simulink model "gpsnoise"  (Simulink 3.00)
settings: Solver=ode45  StartTime=0.0  StopTime=500.0  RelTol=1e-3
libraries: simulink3 x4
settings Model: BooleanDataType=on  RTWOptions="-aEnforceIntegerDowncast=1 -aFoldNonRolledExpr=1 -aInlineInvariantSignals=1 -aInlineParameters=0 -aLocalBlockOutputs=1 -aRollThreshold=5 -aZeroInternalMemoryAtStartup=1 -aZeroExternalMemoryAtStartup=1 -aInitFltsAndDblsToZero=1 -aGenerateReport=0 -aGenCodeOnly=0 -aRTWVerbose=1 -aIncludeHyperlinkInReport=0 -aLaunchReport=0 -aForceParamTrailComments=0 -aGenerateComments=1 -aIgnoreCustomStorageClasses=1 -aIncHierarchyInIds=0 -aMaxRTWIdLen=31 -aShowEliminatedStatements=0 -aPrefixModelToSubsysFcnNames=1 -aIncDataTypeInIds=0 -aInsertBlockDesc=0 -aSimulinkBlockComments=1 -aInlinedPrmAccess=\"Literals\"  -aSuppressErrorStatus=0 -aModelReferenceCompliant=1 -aSupportNonInlinedSFcns=1 -aSupportContinuousTime=1 -aSupportComplex=1 -aSupportNonFinite=1 -aSupportAbsoluteTime=1 -aTargetFcnLib=\"ansi_tfl_tmw.mat\" -aMultiInstanceERTCode=0 -aLogVarNameModifier=\"rt_\" -aIsPILTarget=0 -aCombineOutputUpdateFcns=0 -aGenerateASAP2=0 -aGenerateSampleERTMain=0 -aGenerateFullHeader=1 -aUtilityFuncGeneration=\"Auto\" -aIncludeFileDelimiter=\"Auto\" -aIncludeMdlTerminateFcn=1 -aPurelyIntegerCode=0 -aERTCustomFileBanners=0 -aRTWCAPIStates=0 -aRTWCAPIParams=0 -aRTWCAPISignals=0 -aMatFileLogging=1 -aGenFloatMathFcnCalls=\"ANSI_C\" -aExtModeMexFile=\"ext_comm\" -aExtModeTransport=0 -aExtModeStaticAllocSize=1000000 -aExtModeTesting=0 -aExtModeStaticAlloc=0 -aExtMode=0"  ExtModeTrigMode=normal  ExtModeArmWhenConnect=on  LastModifiedBy=campa

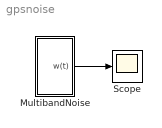
== system gpsnoise ==
  MultibandNoise : Subsystem  mask(Multiband Noise){n=3, power=[2e-5 0.01 0.2 2], time=[0.05 1 10 200], a=2, sd=3587, STime=0.1}
      mask prompts: n "Number Of Channels"; power "Noise Powers"; time "Sample Times (sec)"; a "Filter Cutoff Frequency (rad/sec)"; sd "Base Seed"; STime "Output Sampling Time"
      mask help:
      | This block models multiband noise using four different band limited
      |  white noise blocks, each one with its own power and time scale.
      |  A first order lowpass filter with a selectable cut off frequency is
      |  applied to the last three noises (have a look under the mask).
      |  The output sampling time has to be multiple of the first sample time.
      mask init:
      | n=fix(n);
      | T=time(1);T1=time(2);T2=time(3);T3=time(4);
      | P=power(1);P1=power(2);P2=power(3);P3=power(4);
      mask Help:
      | This block models multiband noise using four different band limited
      |  white noise blocks, each one with its own power and time scale.
      |  A first order lowpass filter with a selectable cut off frequency is
      |  applied to the last three noises (have a look under the mask).
      |  The output sampling time has to be multiple of the first sample time.
  Scope : Scope
      settings: TimeRange=500  YMin=-1  YMax=1  SaveToWorkspace=off  SaveName=ScopeData
  wires:
  MultibandNoise/1(w(t)) -> Scope/1

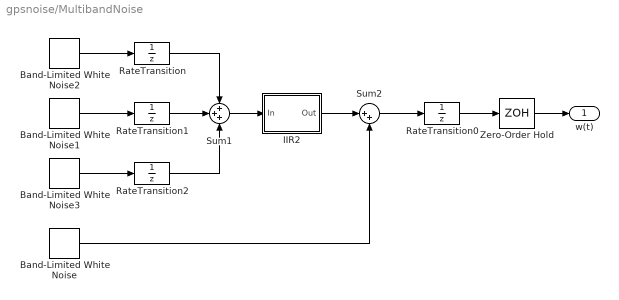
== system gpsnoise/MultibandNoise ==
  Band-Limited White Noise : simulink3/Sources/Band-Limited White Noise  Cov=P*ones(n,1)  Ts=T  seed=sd+[1:n]+0*n
  Band-Limited White Noise1 : simulink3/Sources/Band-Limited White Noise  Cov=P2*ones(n,1)  Ts=T2  seed=sd+[1:n]+2*n
  Band-Limited White Noise2 : simulink3/Sources/Band-Limited White Noise  Cov=P3*ones(n,1)  Ts=T3  seed=sd+[1:n]+1*n
  Band-Limited White Noise3 : simulink3/Sources/Band-Limited White Noise  Cov=P1*ones(n,1)  Ts=T1  seed=sd+[1:n]+3*n
  IIR2 : Subsystem  mask(Discrete Time First Order IIR){ni=n, a=a, x0=0, T=T}
      mask prompts: ni "Number of Channels"; a "Cutoff Frequency (a)"; x0 "Initial Condition"; T "Sample Time"
      mask help:
      | Each channel has the transfer function
      |   (1-exp(-aT))/(1-exp(-aT)(z^-1)) which is a good
      |   (pz-matched) approximation of a/(s+a) if 10*a*T<pi
      mask init:
      | A=[];B=[];C=[];D=[];
      | for i=1:ni,
      | A=[A,zeros(size(A,1),1);zeros(1,size(A,2)),exp(-a*T)];
      | B=[B,zeros(size(B,1),1);zeros(1,size(B,2)),1-exp(-a*T)];
      | C=[C,zeros(size(C,1),1);zeros(1,size(C,2)),exp(-a*T)];
      | D=[D,zeros(size(D,1),1);zeros(1,size(D,2)),1-exp(-a*T)];
      | end
      mask Help:
      | <p>
      |   Each channel has the transfer function
      |   (1-exp(-aT))/(1-exp(-aT)(z^-1)) which is a good
      |   (pz-matched) approximation of a/(s+a) if 10*a*T<pi
      | </p>
      mask Display: dpoly(a,[1 a],'s')
  RateTransition : UnitDelay  X0=0  SampleTime=T3
  RateTransition0 : UnitDelay  X0=0  SampleTime=T
  RateTransition1 : UnitDelay  X0=0  SampleTime=T2
  RateTransition2 : UnitDelay  X0=0  SampleTime=T1
  Sum1 : Sum  Inputs=+++  SaturateOnIntegerOverflow=off
  Sum2 : Sum  Inputs=|++  SaturateOnIntegerOverflow=off
  Zero-Order Hold : ZeroOrderHold  SampleTime=STime
  w(t) : Outport  Port=1
  wires:
  Band-Limited White Noise2/1 -> RateTransition/1
  Band-Limited White Noise1/1 -> RateTransition1/1
  Band-Limited White Noise3/1 -> RateTransition2/1
  Sum1/1 -> IIR2/1(In)
  RateTransition/1 -> Sum1/1
  RateTransition1/1 -> Sum1/2
  RateTransition2/1 -> Sum1/3
  IIR2/1(Out) -> Sum2/1
  Sum2/1 -> RateTransition0/1
  Band-Limited White Noise/1 -> Sum2/2
  RateTransition0/1 -> Zero-Order Hold/1
  Zero-Order Hold/1 -> w(t)/1

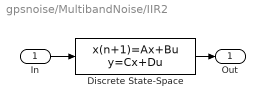
== system gpsnoise/MultibandNoise/IIR2 ==
  In : Inport  Port=1  PortWidth=-1  SampleTime=-1  DataType=auto
      settings: SignalType=auto
  Discrete State-Space : DiscreteStateSpace  A=A  B=B  C=C  D=D  X0=x0  SampleTime=T
  Out : Outport  Port=1
  wires:
  Discrete State-Space/1 -> Out/1
  In/1 -> Discrete State-Space/1
